simulink model "DragModelSeparateRotors"  (R2018b)
settings: Solver=VariableStepAuto  StartTime=0.0  StopTime=10.0  RelTol=1e-3  EnableMultiTasking=on
settings Model: Creator=jban039  LastModifiedBy=jban039
settings DataIOCC: LimitDataPoints=on
settings OptimizationCC: LifeSpan=inf
settings DebuggingCC: AllowSymbolicDim=off  SFUnexpectedBacktrackingDiag=warning  SFNoUnconditionalDefaultTransitionDiag=warning  SFExecutionAtInitializationDiag=none
settings ModelReferenceCC: PropagateSignalLabelsOutOfModel=off
settings SFSimCC: SimUseLocalCustomCode=off
settings RTWCC: RTWUseLocalCustomCode=off
settings CodeAppCC: StateflowObjectComments=on
settings GRTTargetCC: TargetLangStandard=C89/C90 (ANSI)
settings ConfigComp: CovMetricSettings=dw  CovHtmlReporting=on  CovSaveCumulativeToWorkspaceVar=on  CovSaveSingleToWorkspaceVar=on  CovExternalEMLEnable=off

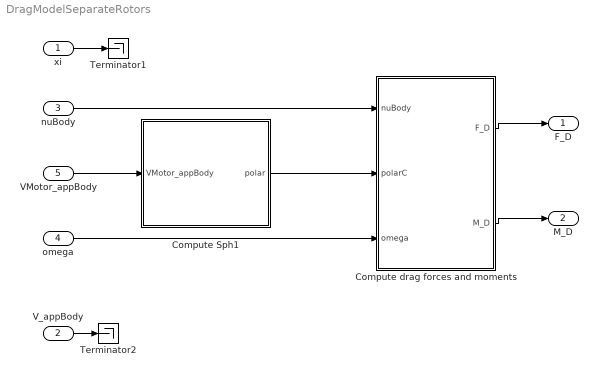
== system DragModelSeparateRotors ==
  xi : Inport  PortDimensions=3
  V_appBody : Inport  Port=2  PortDimensions=3
  nuBody : Inport  Port=3  PortDimensions=3
  omega : Inport  Port=4  PortDimensions=Uav.N_ROTORS
  VMotor_appBody : Inport  Port=5  PortDimensions=[3,4]
  Compute Sph1 : MATLAB Function  TreatAsAtomicUnit=on
  Compute drag forces and moments : MATLAB Function  TreatAsAtomicUnit=on
  Terminator1 : Terminator
  Terminator2 : Terminator
  F_D : Outport
  M_D : Outport  Port=2
  wires:
  Compute drag forces and moments/1(F_D) -> F_D/1
  Compute drag forces and moments/2(M_D) -> M_D/1
  xi/1 -> Terminator1/1
  omega/1 -> Compute drag forces and moments/3(omega)
  nuBody/1 -> Compute drag forces and moments/1(nuBody)
  VMotor_appBody/1 -> Compute Sph1/1(VMotor_appBody)
  Compute Sph1/1(polar) -> Compute drag forces and moments/2(polarC)
  V_appBody/1 -> Terminator2/1

== matlab function DragModelSeparateRotors/Compute drag forces and moments ==
  data: nuBody input; polarC input; omega input; F_D output; M_D output; Uav parameter
function [F_D, M_D] = computeDrag(nuBody, polarC, omega, Uav)
%#codegen

azimuth   = polarC(1,:);
elevation = polarC(2,:);
radius    = polarC(3,:);

% Margin to prevent shattering - doesn't seem to work
% for i = 1:3
%     if ( ( V_appBody(i) > -0.002 ) && ( V_appBody(i) < 0.002 ) )
%         V_appBody(i) = 0;
%     end
% end

% Convert from polar to spherical coordinates
% [ azimuth, elevation, radius ] = cart2sph( V_appBody(1), V_appBody(2), V_appBody(3) );

% elevationAbs = abs(elevation);
% 
% if ( elevationAbs > pi/4 )
%     elevationAbs = pi/4;
% end

% A =  0.0381169670063285+...
%      0.00544289693851381   * elevationAbs + ...
%     -1.40320372862409e-05 * mean( omega ) + ...
%      0.0957929844288627    * elevationAbs^2 + ...
%     -3.68966937291996e-05 * elevationAbs * mean( omega ) + ...
%     -5.12058246754513e-08 * mean( omega ).^2;
% B =  2.26155855608694e-05 + ...
%      2.61717004305892e-05 * elevationAbs + ...
%      2.25793855676601e-06 * mean( omega );

A =  1.691827013696288e-01 + ...
    -1.296810868298392e-01 * cos(-elevation) + ...
    -6.165562917427734e-05 * omega' + ...
     1.745617317423599e-05 * cos(-elevation) .* omega' + ...
     1.587622118174535e-08 * omega'.^2;
B = -2.677662266228434e-01 + ...
     2.538589720234431e-01 * cos(-elevation) + ...
     2.743121165911884e-04 * omega' + ...
     4.813186228167399e-04 * cos(-elevation) .* omega' + ...
     3.930873876708278e-07 * omega'.^2;

% A  = 3.922073463294323e-02 + 3.047871210062095e-02 * abs(eta(2)) + ...
%    -3.963450428543714e-05 * mean( omega );

% B = 2.261558556086950e-05 + 2.617170043058871e-05 * abs(eta(2)) + ...
%    2.257938556766014e-06 * mean( omega );

% % Calculate linear drag force
% f_D = 0.5 * Uav.RHO_AIR * A * radius^2 + ...
%     0.5 * Uav.RHO_AIR * B * radius * mean(omega);
% F_D = zeros(3,1);

f_D = 0.25 * ( 0.5 * Uav.RHO_AIR * A .* radius.^2 + ...
      0.5 * Uav.RHO_AIR * B .* radius );
F_DInd = zeros(3,4);

f_l = 0.25 * ( 0.5 * Uav.RHO_AIR * -( -3.928287694836059e-02 * -elevation + 8.917477120052557e-03) .* radius.^2 );
F_lInd = zeros(3,4);

for i = 1:4
    [ F_DInd(1,i), F_DInd(2,i), F_DInd(3,i) ] = sph2cart( azimuth(i), elevation(i), f_D(:,i) );
    [ F_lInd(1,i), F_lInd(2,i), F_lInd(3,i) ] = sph2cart( azimuth(i), elevation(i) + pi/2, f_l(:,i) );
end

F_D = sum( F_DInd, 2 );
F_l = sum( F_lInd, 2 );

F_D = F_D - F_l;

% Drag moment, applied to independent axes
M_D = 0.5 * Uav.RHO_AIR * Uav.C_DM * ( norm(nuBody) .* nuBody );

== matlab function DragModelSeparateRotors/Compute Sph1 ==
  data: VMotor_appBody input; polar output
function polar  = computeSph(VMotor_appBody)
%#codegen

% Convert from polar to spherical coordinates
radius = zeros(1,4);
elevation = zeros(1,4);
azimuth = zeros(1,4);

for i = 1:length( radius )
    [ azimuth(1,i), elevation(1,i), radius(1,i) ] = ...
        cart2sph( VMotor_appBody(1,i), VMotor_appBody(2,i), VMotor_appBody(3,i) );
end


polar = [azimuth; elevation; radius];
